simulink model "allpassreverb"  (Simulink 7.9)
settings: Solver=FixedStepDiscrete  StartTime=0.0  StopTime=5  RelTol=1e-3
libraries: dspsigops x1, dspvision x1, dspmtrx3 x1, dspsnks4 x1
settings Model: Creator=Arun  LastModifiedBy=ArunKB
settings DebuggingCC: FcnCallInpInsideContextMsg=Use local settings
settings GRTTargetCC: CombineOutputUpdateFcns=off  GRTInterface=on

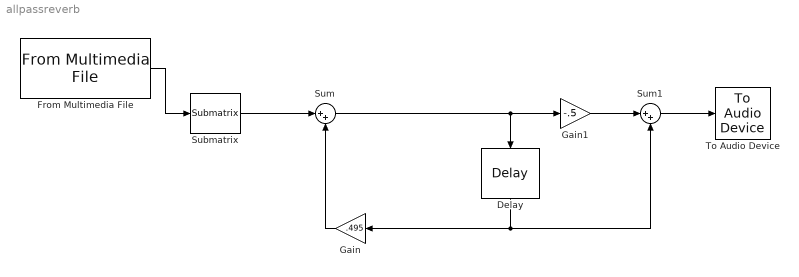
== system allpassreverb ==
  Delay : dspsigops/Delay  InputProcessing=Columns as channels (frame based)  dly_unit=Samples  delay=2500  ic_detail=off  dif_ic_for_ch=off  dif_ic_for_dly=off  ic=0  reset_popup=None
  From Multimedia File : dspvision/From Multimedia File  inputFilename=C:\Users\ArunKB\Documents\MATLAB\reverb\-1 - ElectricGuitarSounds.com.WAV  loop=on  numPlays=1  outputStreams=Audio only  videoDataType=single  audioDataType=double  inheritSampleTime=on  userDefinedSampleTime=1/30  noAudioOutput=off  isIntensityVideo=off  fourcc=RGB  colorVideoFormat=Separate color signals  outputEOF=off  dataOrg=Column-major  audioFrameSize=1  computeAudioFrameSize=off  outSamplingMode=Frame based
  Gain : Gain  Gain=.495
  Gain1 : Gain  Gain=-.5
  Submatrix : dspmtrx3/Submatrix  RowSpan=All rows  RowStartMode=First  RowStartIndex=1  RowEndMode=Last  RowEndIndex=1  ColSpan=One column  ColStartMode=First  ColStartIndex=1  ColEndMode=Last  ColEndIndex=1
  Sum : Sum  Inputs=|++
  Sum1 : Sum  Inputs=|++
  To Audio Device : dspsnks4/To Audio Device  deviceName=Default  inheritSampleRate=on  sampleRate=44100  deviceDatatype=Determine from input data type  autoBufferSize=on  bufferSize=4096  queueDuration=1.0
  wires:
  Submatrix/1 -> Sum/1
  Sum/1 -> Delay/1, Gain1/1
  Gain/1 -> Sum/2
  Delay/1 -> Gain/1, Sum1/2
  Gain1/1 -> Sum1/1
  Sum1/1 -> To Audio Device/1
  From Multimedia File/1 -> Submatrix/1
